simulink model "Real_model"  (R2023b)
settings: Solver=VariableStepAuto  StartTime=0.0  StopTime=T_simulazione  MaxStep=dT  RelTol=1e-3
values from neighbouring files (symbols this model uses):
  dT = 1/f_max    [inizializzazione.m]
  f_max = sensor.d2.freq    [inizializzazione.m]
  f_min = sensor.d2.freq    [inizializzazione.m]
  P0 = [init.q_std_dev(1,1)^2 0 0 0;       0 init.q_std_dev(2,2)^2 0 0;       0 0 init.q_d_std_dev(1,1)^2 0;       0 0 0 init.q_d_std_dev(2,2)^2]    [inizializzazione.m]
  particles0 = mvnrnd (x0_hat, P0, N)    [inizializzazione.m]
  weights0 = 1/N*ones(N,1)    [inizializzazione.m]
  x0_hat = [init.q0(1) init.q0(2) init.q0_d(1) init.q0_d(2)]'    [inizializzazione.m]
undefined symbols (not defined in the file or in its folder): Fext, init, param, param_real, sensor
libraries: simulink x1
settings Model: Creator=jacoc  LastModifiedBy=jacoc

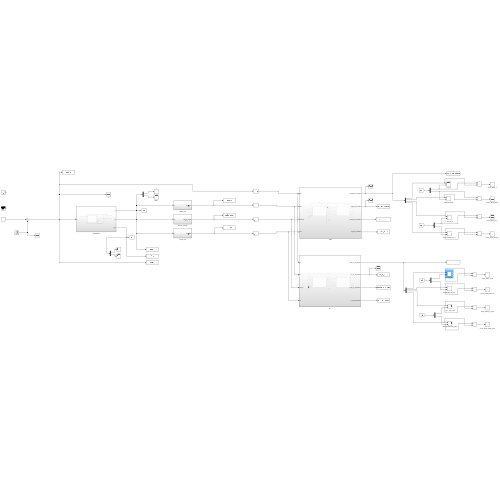
[thumbnail: Simulink's stored preview of the top-level diagram]
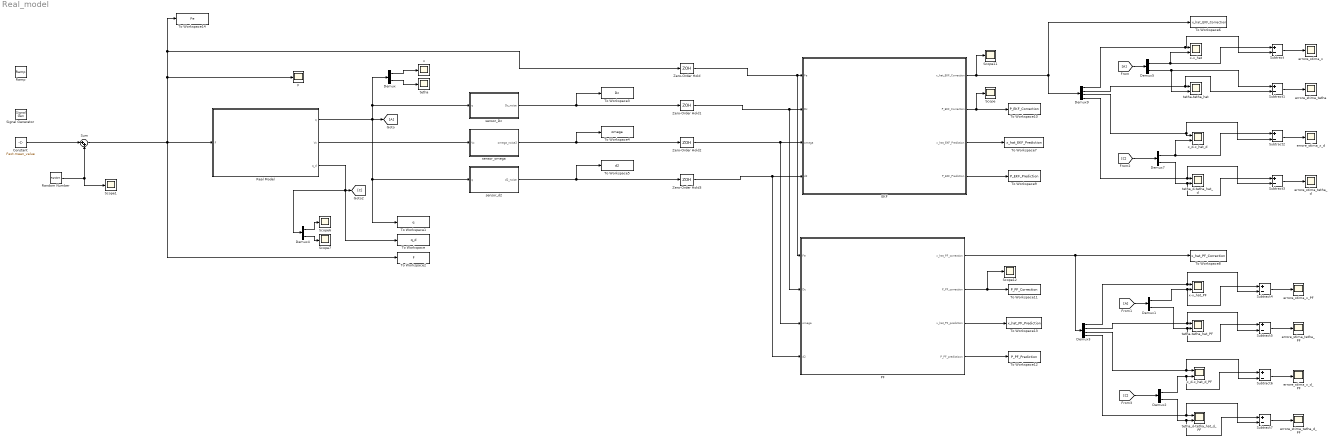
== system Real_model ==
  Constant : Constant  Value=Fext.mean_value
  Demux{,1..2,4..5,7} (6 alike) : Demux  Outputs=2
  Demux3 : Demux
  Demux9 : Demux
  EKF : Subsystem
  F : Scope
  From : From
  From1 : From
  Goto : Goto
  PF : Subsystem
  Ramp : simulink/Sources/Ramp  slope=1  start=0  InitialOutput=0
  Random Number : RandomNumber  Variance=Fext.std_dev^2  Seed=Fext.seed  SampleTime=dT
  Real Model : Subsystem
  Scope{,1,6..7,11..12} (6 alike) : Scope
  Signal Generator : SignalGenerator  Amplitude=200  Frequency=0.1  Units=rad/sec
  Subtract{,1..7} (8 alike) : Sum  Inputs=+-
  Sum : Sum  Inputs=|++
  To Workspace : ToWorkspace  VariableName=q_d  SaveFormat=Timeseries  SampleTime=-1
  To Workspace1 : ToWorkspace  VariableName=q  SaveFormat=Timeseries  SampleTime=-1
  To Workspace10 : ToWorkspace  VariableName=P_EKF_Correction  SaveFormat=Timeseries  SampleTime=-1
  To Workspace11 : ToWorkspace  VariableName=P_PF_Correction  SaveFormat=Timeseries  SampleTime=-1
  To Workspace12 : ToWorkspace  VariableName=P_PF_Prediction  SaveFormat=Timeseries  SampleTime=-1
  To Workspace13 : ToWorkspace  VariableName=x_hat_PF_Prediction  SaveFormat=Timeseries  SampleTime=-1
  To Workspace14 : ToWorkspace  VariableName=Fe  SaveFormat=Timeseries  SampleTime=-1
  To Workspace2 : ToWorkspace  VariableName=F  SaveFormat=Timeseries  SampleTime=-1
  To Workspace3 : ToWorkspace  VariableName=Dc  SaveFormat=Timeseries  SampleTime=-1
  To Workspace4 : ToWorkspace  VariableName=omega  SaveFormat=Timeseries  SampleTime=-1
  To Workspace5 : ToWorkspace  VariableName=d2  SaveFormat=Timeseries  SampleTime=-1
  To Workspace6 : ToWorkspace  VariableName=x_hat_EKF_Correction  SaveFormat=Timeseries  SampleTime=-1
  To Workspace7 : ToWorkspace  VariableName=x_hat_EKF_Prediction  SaveFormat=Timeseries  SampleTime=-1
  To Workspace8 : ToWorkspace  VariableName=x_hat_PF_Correction  SaveFormat=Timeseries  SampleTime=-1
  To Workspace9 : ToWorkspace  VariableName=P_EKF_Prediction  SaveFormat=Timeseries  SampleTime=-1
  Zero-Order Hold{,1..3} (4 alike) : ZeroOrderHold  SampleTime=1/f_max
  errore_stima_tetha : Scope
  errore_stima_tetha_PF : Scope
  errore_stima_tetha_d : Scope
  errore_stima_tetha_d_PF : Scope
  errore_stima_x : Scope
  errore_stima_x_PF : Scope
  errore_stima_x_d : Scope
  errore_stima_x_d_PF : Scope
  sensor_Dc : Subsystem
  sensor_d2 : Subsystem
  sensor_omega : Subsystem
  tetha : Scope
  tetha-tetha_hat : Scope  NumInputPorts=2
  tetha-tetha_hat_PF : Scope  NumInputPorts=2
  tetha_d-tetha_hat_d : Scope  NumInputPorts=2
  tetha_d-tetha_hat_d_PF : Scope  NumInputPorts=2
  x : Scope
  x-x_hat : Scope  NumInputPorts=2
  x-x_hat_PF : Scope  NumInputPorts=2
  x_d-x_hat_d : Scope  NumInputPorts=2
  x_d-x_hat_d_PF : Scope  NumInputPorts=2
  wires:
  Demux/1 -> x/1
  Real Model/2(Vc) -> sensor_omega/1(Vc)
  Demux4/1 -> Scope6/1
  Demux4/2 -> Scope7/1
  Demux/2 -> tetha/1
  Real Model/3(q_d) -> Demux4/1, [C], To Workspace/1
  Real Model/1(q) -> Goto/1, sensor_Dc/1(q), Demux/1, sensor_d2/1(q), To Workspace1/1
  Subtract6/1 -> errore_stima_x_d_PF/1
  Demux1/1 -> Subtract4/1, x-x_hat_PF/2
  Subtract7/1 -> errore_stima_tetha_d_PF/1
  Demux5/1 -> x-x_hat/2, Subtract/1
  Subtract4/1 -> errore_stima_x_PF/1
  Demux5/2 -> tetha-tetha_hat/2, Subtract1/1
  [C] -> Demux2/1
  Demux9/2 -> Subtract1/2, tetha-tetha_hat/1
  Subtract1/1 -> errore_stima_tetha/1
  sensor_d2/1(d2_noise) -> Zero-Order Hold3/1, To Workspace5/1
  Subtract5/1 -> errore_stima_tetha_PF/1
  Zero-Order Hold3/1 -> EKF/4(d2), PF/4(d2)
  EKF/4(P_EKF_Prediction) -> To Workspace9/1
  PF/2(P_PF_correction) -> Scope12/1, To Workspace11/1
  Subtract2/1 -> errore_stima_x_d/1
  Subtract3/1 -> errore_stima_tetha_d/1
  Subtract/1 -> errore_stima_x/1
  PF/4(P_PF_predictioon) -> To Workspace12/1
  Demux3/4 -> tetha_d-tetha_hat_d_PF/1, Subtract7/2
  PF/3(x_hat_PF_prediction) -> To Workspace13/1
  From1/1 -> Demux1/1
  Demux2/2 -> tetha_d-tetha_hat_d_PF/2, Subtract7/1
  Demux2/1 -> x_d-x_hat_d_PF/2, Subtract6/1
  PF/1(x_hat_PF_correction) -> To Workspace8/1, Demux3/1
  Demux3/1 -> Subtract4/2, x-x_hat_PF/1
  Demux7/2 -> Subtract3/1, tetha_d-tetha_hat_d/2
  Demux1/2 -> Subtract5/1, tetha-tetha_hat_PF/2
  Demux7/1 -> x_d-x_hat_d/2, Subtract2/1
  Zero-Order Hold/1 -> PF/1(Fe), EKF/1(Fe)
  EKF/1(x_hat_EKF_Correction) -> Demux9/1, To Workspace6/1, Scope11/1
  Demux9/4 -> Subtract3/2, tetha_d-tetha_hat_d/1
  EKF/3(x_hat_EKF_Prediction) -> To Workspace7/1
  Demux3/3 -> x_d-x_hat_d_PF/1, Subtract6/2
  Demux9/1 -> x-x_hat/1, Subtract/2
  EKF/2(P_EKF_Correction) -> To Workspace10/1, Scope/1
  Demux3/2 -> Subtract5/2, tetha-tetha_hat_PF/1
  Demux9/3 -> x_d-x_hat_d/1, Subtract2/2
  [C] -> Demux7/1
  Zero-Order Hold2/1 -> EKF/3(omega), PF/3(omega)
  sensor_omega/1(omega_noise2) -> Zero-Order Hold2/1, To Workspace4/1
  Sum/1 -> Zero-Order Hold/1, To Workspace14/1, F/1, To Workspace2/1, Real Model/1(F)
  From/1 -> Demux5/1
  sensor_Dc/1(Dc_noise) -> Zero-Order Hold1/1, To Workspace3/1
  Zero-Order Hold1/1 -> EKF/2(Dc), PF/2(Dc)
  Constant/1 -> Sum/1
  Random Number/1 -> Scope1/1, Sum/2

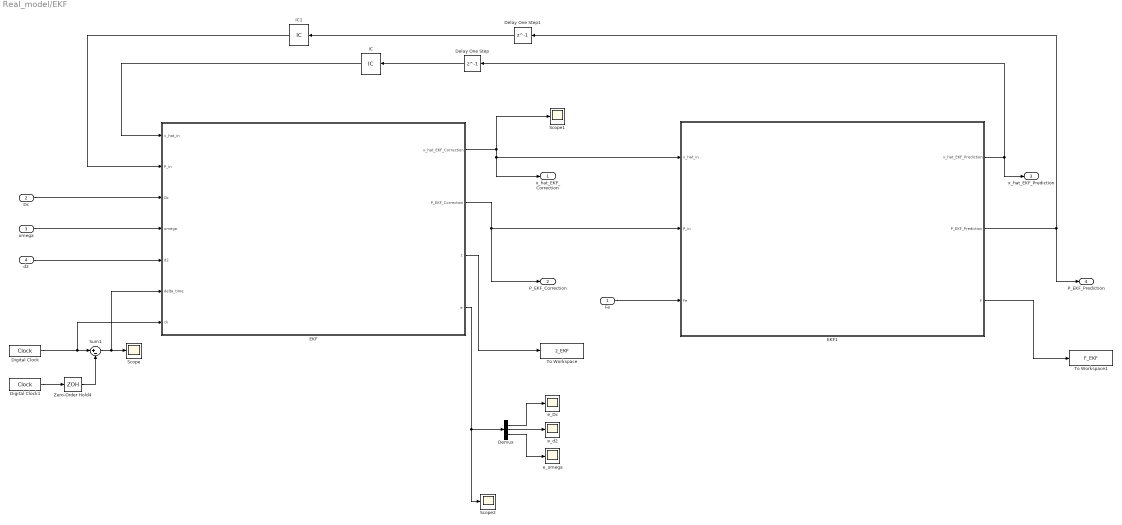
== system Real_model/EKF ==
  Fe : Inport
  Dc : Inport  Port=2
  omega : Inport  Port=3
  d2 : Inport  Port=4
  Delay One Step : Delay  DelayLength=1
  Delay One Step1 : Delay  DelayLength=1
  Demux : Demux  Outputs=3
  Digital Clock : DigitalClock  SampleTime=1/f_max
  Digital Clock1 : DigitalClock  SampleTime=1/f_min
  EKF : MATLAB Function  TreatAsAtomicUnit=on
  EKF1 : MATLAB Function  TreatAsAtomicUnit=on
  IC : InitialCondition  Value=x0_hat
  IC1 : InitialCondition  Value=P0
  Scope : Scope
  Scope1 : Scope
  Scope2 : Scope
  Sum1 : Sum  Inputs=|+-
  To Workspace : ToWorkspace  VariableName=z_EKF  SaveFormat=Timeseries  SampleTime=-1
  To Workspace1 : ToWorkspace  VariableName=F_EKF  SaveFormat=Timeseries  SampleTime=-1
  Zero-Order Hold4 : ZeroOrderHold  SampleTime=1/f_max
  e_Dc : Scope
  e_d2 : Scope
  e_omega : Scope
  x_hat_EKF_Correction : Outport
  P_EKF_Correction : Outport  Port=2
  x_hat_EKF_Prediction : Outport  Port=3
  P_EKF_Prediction : Outport  Port=4
  wires:
  Digital Clock/1 -> EKF/7(ck), Sum1/1
  Digital Clock1/1 -> Zero-Order Hold4/1
  Sum1/1 -> Scope/1, EKF/6(delta_time)
  Zero-Order Hold4/1 -> Sum1/2
  Delay One Step/1 -> IC/1
  Delay One Step1/1 -> IC1/1
  EKF/1(x_hat_EKF_Correction) -> EKF1/1(x_hat_in), x_hat_EKF_Correction/1, Scope1/1
  EKF/2(P_EKF_Correction) -> EKF1/2(P_in), P_EKF_Correction/1
  Dc/1 -> EKF/3(Dc)
  omega/1 -> EKF/4(omega)
  d2/1 -> EKF/5(d2)
  Fe/1 -> EKF1/3(Fe)
  EKF1/1(x_hat_EKF_Prediction) -> x_hat_EKF_Prediction/1, Delay One Step/1
  EKF1/2(P_EKF_Prediction) -> P_EKF_Prediction/1, Delay One Step1/1
  IC1/1 -> EKF/2(P_in)
  IC/1 -> EKF/1(x_hat_in)
  EKF/3(z) -> To Workspace/1
  EKF/4(e) -> Scope2/1, Demux/1
  Demux/1 -> e_Dc/1
  Demux/2 -> e_d2/1
  Demux/3 -> e_omega/1
  EKF1/3(F) -> To Workspace1/1

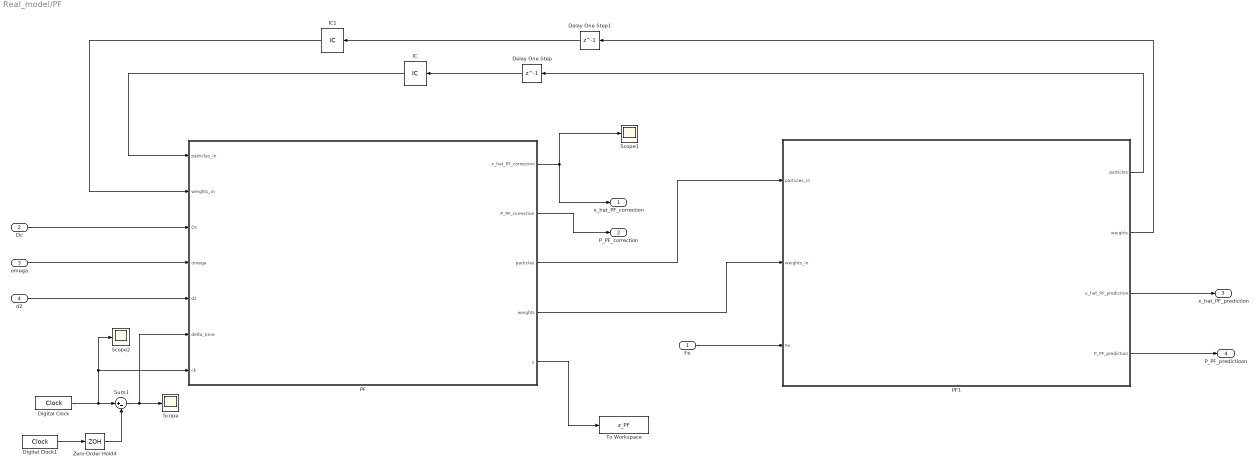
== system Real_model/PF ==
  Fe : Inport
  Dc : Inport  Port=2
  omega : Inport  Port=3
  d2 : Inport  Port=4
  Delay One Step : Delay  DelayLength=1
  Delay One Step1 : Delay  DelayLength=1
  Digital Clock : DigitalClock  SampleTime=1/f_max
  Digital Clock1 : DigitalClock  SampleTime=1/f_min
  IC : InitialCondition  Value=particles0
  IC1 : InitialCondition  Value=weights0
  PF : MATLAB Function  TreatAsAtomicUnit=on
  PF1 : MATLAB Function  TreatAsAtomicUnit=on
  Scope : Scope
  Scope1 : Scope
  Scope2 : Scope
  Sum1 : Sum  Inputs=|+-
  To Workspace : ToWorkspace  VariableName=z_PF  SaveFormat=Timeseries  SampleTime=-1
  Zero-Order Hold4 : ZeroOrderHold  SampleTime=1/f_max
  x_hat_PF_correction : Outport
  P_PF_correction : Outport  Port=2
  x_hat_PF_prediction : Outport  Port=3
  P_PF_predictioon : Outport  Port=4
  wires:
  Digital Clock/1 -> Scope2/1, PF/7(ck), Sum1/1
  Digital Clock1/1 -> Zero-Order Hold4/1
  Sum1/1 -> Scope/1, PF/6(delta_time)
  Zero-Order Hold4/1 -> Sum1/2
  Delay One Step/1 -> IC/1
  Delay One Step1/1 -> IC1/1
  PF/1(x_hat_PF_correction) -> x_hat_PF_correction/1, Scope1/1
  PF/2(P_PF_correction) -> P_PF_correction/1
  Dc/1 -> PF/3(Dc)
  omega/1 -> PF/4(omega)
  d2/1 -> PF/5(d2)
  Fe/1 -> PF1/3(Fe)
  PF1/1(particles) -> Delay One Step/1
  PF1/2(weights) -> Delay One Step1/1
  IC1/1 -> PF/2(weights_in)
  IC/1 -> PF/1(particles_in)
  PF/3(particles) -> PF1/1(particles_in)
  PF/4(weights) -> PF1/2(weights_in)
  PF/5(z) -> To Workspace/1
  PF1/4(P_PF_prediction) -> P_PF_predictioon/1
  PF1/3(x_hat_PF_prediction) -> x_hat_PF_prediction/1

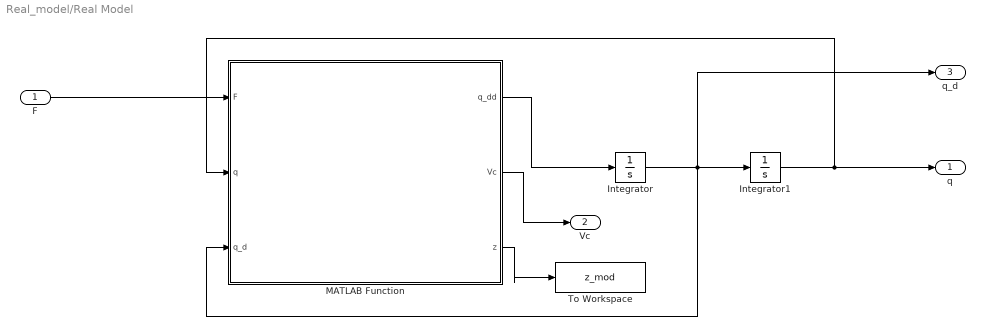
== system Real_model/Real Model ==
  F : Inport
  Integrator : Integrator  InitialCondition=init.real_q0_d
  Integrator1 : Integrator  InitialCondition=init.real_q0
  MATLAB Function : MATLAB Function  TreatAsAtomicUnit=on
  To Workspace : ToWorkspace  VariableName=z_mod  SaveFormat=Timeseries  SampleTime=-1
  q : Outport
  Vc : Outport  Port=2
  q_d : Outport  Port=3
  wires:
  Integrator/1 -> q_d/1, MATLAB Function/3(q_d), Integrator1/1
  MATLAB Function/1(q_dd) -> Integrator/1
  Integrator1/1 -> q/1, MATLAB Function/2(q)
  F/1 -> MATLAB Function/1(F)
  MATLAB Function/2(Vc) -> Vc/1
  MATLAB Function/3(z) -> To Workspace/1

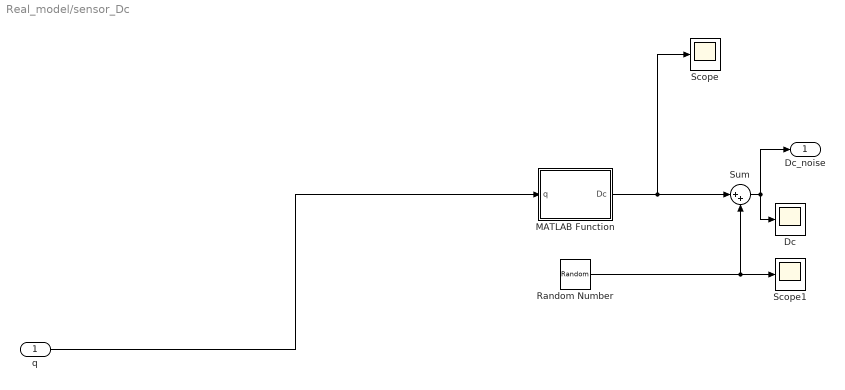
== system Real_model/sensor_Dc ==
  q : Inport
  Dc : Scope
  MATLAB Function : MATLAB Function  TreatAsAtomicUnit=on  SystemSampleTime=1/sensor.Dc.freq
  Random Number : RandomNumber  Variance=sensor.Dc.std_dev^2  Seed=sensor.Dc.seed  SampleTime=1/sensor.Dc.freq
  Scope : Scope
  Scope1 : Scope
  Sum : Sum  Inputs=|++
  Dc_noise : Outport
  wires:
  Random Number/1 -> Scope1/1, Sum/2
  Sum/1 -> Dc_noise/1, Dc/1
  MATLAB Function/1(Dc) -> Sum/1, Scope/1
  q/1 -> MATLAB Function/1(q)

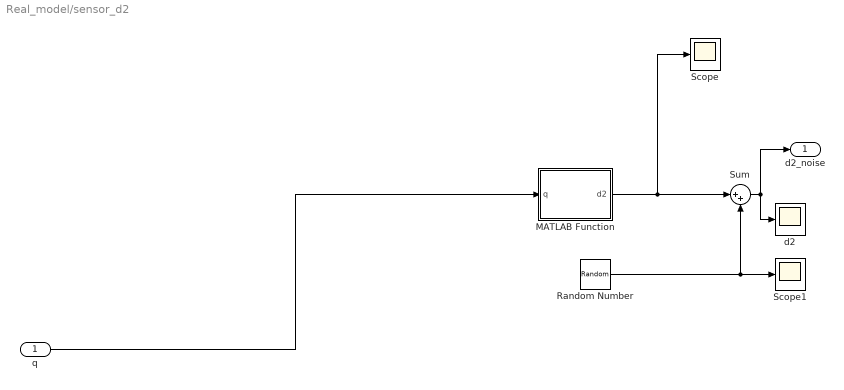
== system Real_model/sensor_d2 ==
  q : Inport
  MATLAB Function : MATLAB Function  TreatAsAtomicUnit=on  SystemSampleTime=1/sensor.d2.freq
  Random Number : RandomNumber  Variance=sensor.d2.std_dev^2  Seed=sensor.d2.seed  SampleTime=1/sensor.d2.freq
  Scope : Scope
  Scope1 : Scope
  Sum : Sum  Inputs=|++
  d2 : Scope
  d2_noise : Outport
  wires:
  Random Number/1 -> Scope1/1, Sum/2
  Sum/1 -> d2_noise/1, d2/1
  MATLAB Function/1(d2) -> Sum/1, Scope/1
  q/1 -> MATLAB Function/1(q)

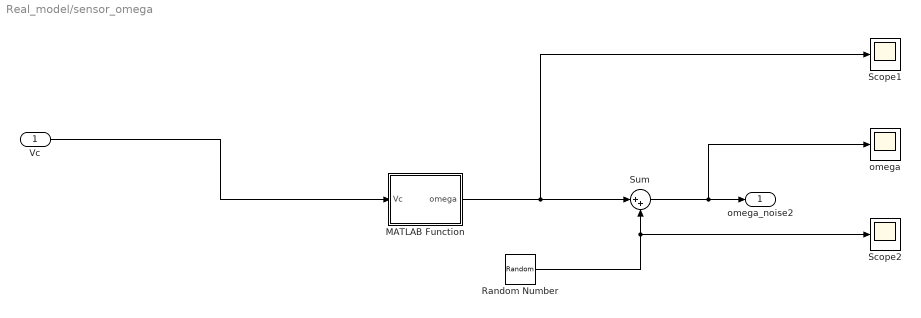
== system Real_model/sensor_omega ==
  Vc : Inport
  MATLAB Function : MATLAB Function  TreatAsAtomicUnit=on  SystemSampleTime=1/sensor.omega.freq
  Random Number : RandomNumber  Variance=sensor.omega.std_dev^2  Seed=sensor.omega.seed  SampleTime=1/sensor.omega.freq  VectorParams1D=off
  Scope1 : Scope
  Scope2 : Scope
  Sum : Sum  Inputs=|++
  omega : Scope
  omega_noise2 : Outport
  wires:
  Random Number/1 -> Scope2/1, Sum/2
  MATLAB Function/1(omega) -> Scope1/1, Sum/1
  Vc/1 -> MATLAB Function/1(Vc)
  Sum/1 -> omega/1, omega_noise2/1

== matlab function Real_model/PF/PF ==
  data: particles_in input; weights_in input; x_hat_PF_correction output; Dc input; omega input; d2 input; param parameter; sensor parameter; Fext parameter; delta_time input; P_PF_correction output; ck input; particles output; weights output; z output
function [ x_hat_PF_correction, P_PF_correction, particles, weights, z]  = Correzione (particles_in, weights_in, Dc, omega, d2, param, sensor, Fext, delta_time, ck)

M = param.M;   
J = param.J;    
Ca = param.Ca;     
L = param.L;       
l = param.l;     
h = param.h; 
g = param.g;
r = param.r;

particles = particles_in;
weights = weights_in;

likelyhood_for_particles = zeros(size(particles,1),1);                                      % inizializzo la stima di massima verosimiglianza

%% correzione
if (delta_time <= 0) && (ck ~= 0)

    for i = 1:size(particles,1)
        likelyhood_Dc = normpdf(Dc - particles(i,1) + (l+r)*sin(particles(i,2)),...         % calcolo la verosimiglianza per ogni sensore per una singola particella
                        0 , sensor.Dc.std_dev^2);  
        likelyhood_d2 = normpdf (d2 + (L-l-r)*sin(particles(i,2)), 0 , sensor.d2.std_dev^2);
        likelyhood_omega = normpdf(omega - particles(i,3)/r + ...
                           (l+r)/r*particles(i,4)*cos(particles(i,2)), 0 , sensor.Dc.std_dev^2);

        likelyhood_for_particles(i,1) = likelyhood_Dc*likelyhood_d2*likelyhood_omega;       % verosimiglianza totale di una particella
    end
    
    weights = (weights.*likelyhood_for_particles)/sum(weights.*likelyhood_for_particles);   % ricalcolo i  delle particelle e li normalizzo
    
    % calcolo la stima e la matrice di covarianza con le particelle e i pesi (anche se non è avvenuta la correzione)
    x_hat_PF_correction = particles'*weights;
    P_PF_correction = zeros(4);
    for i=1:size(particles,1)
    P_PF_correction = P_PF_correction + weights(i)*...
                      (particles(i,1:4)' - x_hat_PF_correction)*...
                      (particles(i,1:4)' - x_hat_PF_correction)';
    end
    %% ricampionamento
    s = cumsum(weights);                                                                    % genero il vettore dei pesi
    epsilon = [0.01 0.001 0.002 0.002];                                                         % vettore che serve per generare campioni diversi
    new_particles = zeros(size(particles));
    
    for j = 1:size(particles,1)
        u = rand(1);                                                                        % numero casuale per pescare casualmente nel vettore s
        csi = epsilon.*randn(1,4);                                                          % genero scostamento casuale della nuova particella
        i = find(s>=u,1,'first');                                                           % trovo l'indice della particella con il peso nel vettore s 
        new_particles(j,:) = particles(i,:) + csi;                                          % genero la nuova particella
    end
    new_weights = 1/size(weights,1) * ones(size(weights,1),1);                              % formatto i pesi a 1/N

    particles = new_particles;                      
    weights = new_weights;  
else
    % calcolo la stima e la matrice di covarianza con le particelle e i pesi (anche se non è avvenuta la correzione)
    x_hat_PF_correction = particles'*weights;
    P_PF_correction = zeros(4);
    for i=1:size(particles,1)
    P_PF_correction = P_PF_correction + weights(i)*...
                      (particles(i,1:4)' - x_hat_PF_correction)*...
                      (particles(i,1:4)' - x_hat_PF_correction)';
    end
end
z = L*cos(x_hat_PF_correction(2));                                                          % variabile usata per il plot

== matlab function Real_model/PF/PF1 ==
  data: particles_in input; weights_in input; Fe input; particles output; param parameter; sensor parameter; Fext parameter; weights output; dT parameter; x_hat_PF_prediction output; P_PF_prediction output
function [particles, weights, x_hat_PF_prediction, P_PF_prediction] = Predizione (particles_in, weights_in, Fe, param, sensor, Fext, dT)

M = param.M;   
J = param.J;    
Ca = param.Ca;     
L = param.L;       
l = param.l;     
h = param.h; 
g = param.g;
r = param.r;


particles = zeros (size(particles_in));
weights = weights_in;
Q = Fext.std_dev^2;                                         % incertezza ingresso

R = [sensor.Dc.std_dev^2 0 0;...                            % matrice incertezze dei sensori
     0 sensor.d2.std_dev^2 0;...
     0 0 sensor.omega.std_dev^2];

%% predizione
% calcolo le particelle tramite le equazioni nella forma di stato
for i = 1:size(particles,1)
    Wf = mvnrnd (0 , Q);
    particles(i,1) = particles_in(i,1) + dT*particles_in(i,3);
    particles(i,2) = particles_in(i,2) + dT*particles_in(i,4);
    particles(i,3) = (1 - dT*Ca/M)*particles_in(i,3) + (dT*Ca*(l+r)/M)*particles_in(i,4)*cos(particles_in(i,2)) + (dT*(Fe+Wf)/M);
    particles(i,4) = (1 - dT*Ca*((l+r)^2)/J*(cos(particles_in(i,2))^2))*particles_in(i,4) - (dT*M*g*(l+r)/J)*sin(particles_in(i,2)) + dT/J*(Ca*(l+r)*particles_in(i,3) - (Fe+Wf)*L)*cos(particles_in(i,2));
    
end
% calcolo le stime predette da mandare in uscita
 x_hat_PF_prediction = particles'*weights;
 P_PF_prediction = zeros(4);
 for i=1:size(particles,1)
     P_PF_prediction = P_PF_prediction + weights(i)*(particles(i,1:4)' - x_hat_PF_prediction)*(particles(i,1:4)' - x_hat_PF_prediction)';
 end

== matlab function Real_model/sensor_Dc/MATLAB Function ==
  data: q input; Dc output; param parameter
function Dc = calcolo_Dc(q,param)

l = param.l;
r=param.r;

Dc = q(1) - (l+r)*sin(q(2));

== matlab function Real_model/Real Model/MATLAB Function ==
  data: F input; q input; q_dd output; q_d input; param parameter; Vc output; z output; param_real parameter
function [q_dd,Vc,z] = fcn(F,q,q_d, param, param_real)

M = param_real.M;   
J = param_real.J;    
Ca = param_real.Ca;     
L = param.L;       
l = param.l;     
h = param.h; 
g = param.g;
r = param.r;

z = L*cos(q(2));

Vc = q_d(1) - (l+r)*q_d(2)*cos(q(2));                                       %velocità del punto C di contatto tra la puleggia ed il cavo di sostegno

x_dd = (-Ca*Vc + F)/M;                                                      %prima equazione cardinale

tetha_dd = (-M*g*(l+r)*sin(q(2)) + Ca*(l+r)*Vc*cos(q(2)) - F*L*cos(q(2)))/J;    %seconda cardinale scritta rispetto al baricentro

q_dd = [x_dd; tetha_dd];

%NOTA:forza di attrito viscoso agisce sul centro della  puleggia

== matlab function Real_model/EKF/EKF ==
  data: x_hat_in input; P_in input; x_hat_EKF_Correction output; Dc input; omega input; d2 input; param parameter; sensor parameter; Fext parameter; delta_time input; P_EKF_Correction output; ck input; z output; e output
function [ x_hat_EKF_Correction, P_EKF_Correction, z, e]  = Correzione (x_hat_in, P_in, Dc, omega, d2, param, sensor, Fext, delta_time, ck)

M = param.M;   
J = param.J;    
Ca = param.Ca;     
L = param.L;       
l = param.l;     
h = param.h; 
g = param.g;
r = param.r;
Dc_std_dev = sensor.Dc.std_dev;
d2_std_dev = sensor.d2.std_dev;
omega_std_dev = sensor.omega.std_dev;

x_hat_EKF_Correction = x_hat_in;

% P = [init.q_std_dev(1)^2 0 0 0;...                        % incertezza iniziale
%      0 init.q_std_dev(2)^2 0 0;...
%      0 0 init.q_d_std_dev(1)^2 0;...
%      0 0 0 init.q_d_std_dev(2)^2];
P_EKF_Correction = P_in;

Q = Fext.std_dev^2;                                         % incertezza ingresso

R = [Dc_std_dev^2 0 0;...                                   % matrice incertezze dei sensori
     0 d2_std_dev^2 0;...
     0 0 omega_std_dev^2];

e = zeros(3,1);

%% correzione
if (delta_time <= 0) && (ck ~= 0)                           % algoritmo di scelta di correzione
    
    % Innovazione                                                 
    e(1) = Dc - ( x_hat_EKF_Correction(1) - (l+r)*sin(x_hat_EKF_Correction(2)) );
    e(2) = d2 + ( (L-l-r)*sin(x_hat_EKF_Correction(2)) );
    e(3) = omega - ( x_hat_EKF_Correction(3) - (l+r)*x_hat_EKF_Correction(4)*cos(x_hat_EKF_Correction(2)) )/r;

    H = [1    -(l+r)*cos(x_hat_EKF_Correction(2))                          0                    0                   ;...
         0    -(L-l-r)*cos(x_hat_EKF_Correction(2))                        0                    0                   ;...
         0 ((l+r)*x_hat_EKF_Correction(4)*sin(x_hat_EKF_Correction(2)))/r 1/r -(l+r)/r*cos(x_hat_EKF_Correction(2))];

    %M = eye(3);                                            % dato che è l'identità non lo consideriamo nelle formule successive
                                                            
    S = H*P_EKF_Correction*H' + R;                          % Covarianza innovazione
    Lk = P_EKF_Correction*H'/S;                             % Guadagno di correzione

    % calcolo la stima e la matrice di covarianza corretta
    x_hat_EKF_Correction = x_hat_EKF_Correction + Lk*e;
    P_EKF_Correction = P_EKF_Correction - Lk*S*Lk';
end

z = L*cos(x_hat_EKF_Correction(2));                         %variabile usata per il plot

== matlab function Real_model/sensor_omega/MATLAB Function ==
  data: Vc input; omega output; param parameter
function omega = fcn(Vc, param)

omega = Vc/param.r;

== matlab function Real_model/sensor_d2/MATLAB Function ==
  data: q input; d2 output; param parameter
function d2 = calcolo_d2(q,param)

l = param.l;
L = param.L;
r=param.r;

d2 = -(L-l-r)*sin(q(2));                                                      %distanza orizzontale tra il punto di aggancio sul cavo di trascinamento e C

== matlab function Real_model/EKF/EKF1 ==
  data: x_hat_in input; P_in input; Fe input; x_hat_EKF_Prediction output; param parameter; sensor parameter; Fext parameter; P_EKF_Prediction output; dT parameter; F output
function [x_hat_EKF_Prediction, P_EKF_Prediction,F] = Predizione (x_hat_in, P_in, Fe, param, sensor, Fext, dT)

M = param.M;   
J = param.J;    
Ca = param.Ca;     
L = param.L;       
l = param.l;     
h = param.h; 
g = param.g;
r = param.r;


x_hat_EKF_Prediction = x_hat_in;

% P = [init.q_std_dev(1)^2 0 0 0;...                                                    % incertezza iniziale
%      0 init.q_std_dev(2)^2 0 0;...
%      0 0 init.q_d_std_dev(1)^2 0;...
%      0 0 0 init.q_d_std_dev(2)^2];
P_EKF_Prediction = P_in;

Q = Fext.std_dev^2;                                                                     % incertezza ingresso

%% predizione
x_hat_EKF_Prediction(1) = x_hat_EKF_Prediction(1) + dT*x_hat_EKF_Prediction(3);         % calcolo la stima predetta
x_hat_EKF_Prediction(2) = x_hat_EKF_Prediction(2) + dT*x_hat_EKF_Prediction(4);
x_hat_EKF_Prediction(3) = (1 - dT*Ca/M)*x_hat_EKF_Prediction(3) + ...
                          (dT*Ca*(l+r)/M)*x_hat_EKF_Prediction(4)*...
                          cos(x_hat_EKF_Prediction(2)) + (dT*Fe/M);
x_hat_EKF_Prediction(4) = (1 - dT*Ca*((l+r)^2)/J*(cos(x_hat_EKF_Prediction(2))^2))*...
                          x_hat_EKF_Prediction(4) - (dT*M*g*(l+r)/J)*sin(x_hat_EKF_Prediction(2))...
                          + dT/J*(Ca*(l+r)*x_hat_EKF_Prediction(3) - Fe*L)*cos(x_hat_EKF_Prediction(2));


F = [1 ...
     0 ...
     dT ...
     0;... 
     0 ...
     1 ...
     0 ...
     dT;...
     0 ...
     -(dT*Ca*(l+r)/M)*x_hat_EKF_Prediction(4)*sin(x_hat_EKF_Prediction(2)) ...
     1-dT*Ca/M ...
     (dT*Ca*(l+r)/M)*cos(x_hat_EKF_Prediction(2));...
     0 ...
     dT/J*( -M*g*(l+r)*cos(x_hat_EKF_Prediction(2)) - Ca*(l+r)*x_hat_EKF_Prediction(3)*sin(x_hat_EKF_Prediction(2)) + Ca*((l+r)^2)*x_hat_EKF_Prediction(4)*cos(x_hat_EKF_Prediction(2))*sin(x_hat_EKF_Prediction(2)) + Fe*L*sin(x_hat_EKF_Prediction(2))) ...
     (dT/J*Ca*(l+r)*cos(x_hat_EKF_Prediction(2))) ...
     (1 - dT*Ca*((l+r)^2)/J*(cos(x_hat_EKF_Prediction(2))^2))];

D = [0 0 dT/M -dT*L/J*cos(x_hat_EKF_Prediction(2))];

P_EKF_Prediction = F*P_EKF_Prediction*F' + D*Q*D';                                      % calcolo la matrice di covarianza predetta
